simulink model "msdMultipleBuildingSoln"  (R2020b)
settings: Solver=VariableStepAuto  StartTime=0.0  StopTime=200  RelTol=1e-6
undefined symbols (not defined in the file): c, k, m, n, x_0, x_dot_0
settings Model: Creator=Rocksmithed  LastModifiedBy=Rocksmithed
settings DataIOCC: SaveFormat=Array
settings HardwareCC: TargetBitPerPointer=64  TargetBitPerSizeT=64  TargetBitPerPtrDiffT=64  TargetLongLongMode=on  TargetIntDivRoundTo=Zero  TargetEndianess=LittleEndian  TargetWordSize=64  TargetHWDeviceType=MATLAB Host  ProdEqTarget=off
settings RTWCC: Description=Rapid Simulation Target  SystemTargetFile=rsim.tlc  TemplateMakefile=rsim_default_tmf
settings RSimTargetCC: TargetLangStandard=C99 (ISO)

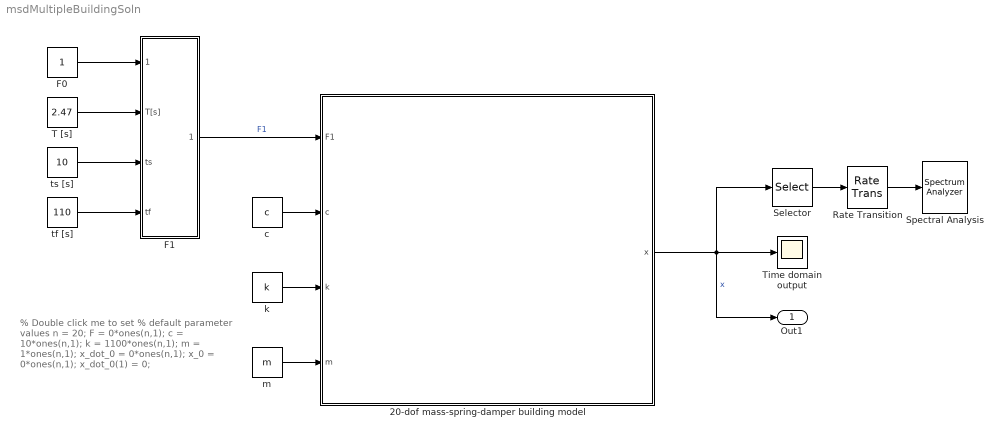
== system msdMultipleBuildingSoln ==
  note: % Double click me to set
      | % default parameter values
      | n = 20;
      | F = 0*ones(n,1);
      | c = 10*ones(n,1);
      | k = 1100*ones(n,1);
      | m = 1*ones(n,1);
      | x_dot_0 = 0*ones(n,1);
      | x_0 = 0*ones(n,1);
      | x_dot_0(1) = 0;
  20-dof mass-spring-damper building model : Subsystem  mask{x0_mask=x_0, x_dot_0_mask=x_dot_0}
      mask prompts: x0_mask "x0"; x_dot_0_mask "x_dot_0"
      mask Display: image('$imagefile'); % Use "Edit Image" on toolstrip to change.
  F0 : Constant
  F1 : Subsystem
  Rate Transition : RateTransition  OutPortSampleTime=0.05
  Selector : Selector  InputPortWidth=n  IndexOptions=Index vector (dialog)  Indices=20  OutputSizes=1
  Spectral Analysis : SpectrumAnalyzer
  T [s] : Constant  Value=2.47
  Time domain output : Scope
  c : Constant  Value=c
  k : Constant  Value=k
  m : Constant  Value=m
  tf [s] : Constant  Value=110
  ts [s] : Constant  Value=10
  Out1 : Outport
  wires:
  Selector/1 -> Rate Transition/1
  Rate Transition/1 -> Spectral Analysis/1
  20-dof mass-spring-damper building model/1(x) -> Selector/1, Out1/1, Time domain output/1  "x"
  c/1 -> 20-dof mass-spring-damper building model/2(c)
  k/1 -> 20-dof mass-spring-damper building model/3(k)
  m/1 -> 20-dof mass-spring-damper building model/4(m)
  tf [s]/1 -> F1/4(tf)
  T [s]/1 -> F1/2(T[s])
  ts [s]/1 -> F1/3(ts)
  F0/1 -> F1/1(F0 [N])
  F1/1(Out1) -> 20-dof mass-spring-damper building model/1(F1)  "F1"

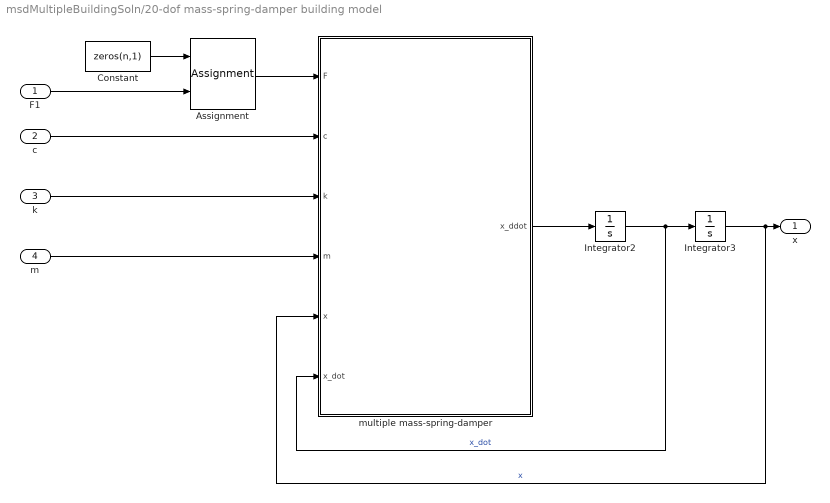
== system msdMultipleBuildingSoln/20-dof mass-spring-damper building model ==
  F1 : Inport
  c : Inport  Port=2
  k : Inport  Port=3
  m : Inport  Port=4
  Assignment : Assignment  DiagnosticForDimensions=Warning  IndexOptions=Index vector (dialog)  Indices=1  OutputSizes=1
  Constant : Constant  Value=zeros(n,1)
  Integrator2 : Integrator  InitialCondition=x_dot_0_mask
  Integrator3 : Integrator  InitialCondition=x0_mask
  multiple mass-spring-damper : MATLAB Function  TreatAsAtomicUnit=on
  x : Outport
  wires:
  k/1 -> multiple mass-spring-damper/3(k)
  Integrator2/1 -> multiple mass-spring-damper/6(x_dot), Integrator3/1  "x_dot"
  Integrator3/1 -> multiple mass-spring-damper/5(x), x/1  "x"
  multiple mass-spring-damper/1(x_ddot) -> Integrator2/1
  c/1 -> multiple mass-spring-damper/2(c)
  m/1 -> multiple mass-spring-damper/4(m)
  F1/1 -> Assignment/2
  Constant/1 -> Assignment/1
  Assignment/1 -> multiple mass-spring-damper/1(F)

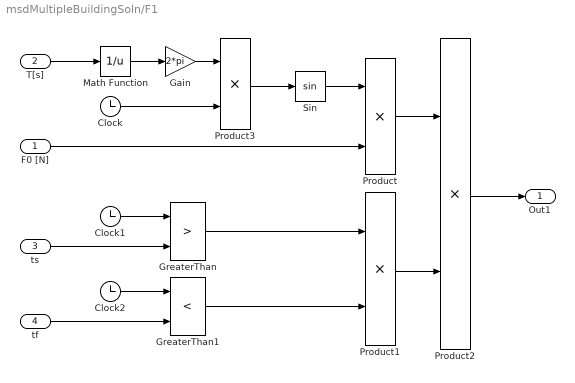
== system msdMultipleBuildingSoln/F1 ==
  F0 [N] : Inport
  T[s] : Inport  Port=2
  ts : Inport  Port=3
  tf : Inport  Port=4
  Clock : Clock
  Clock1 : Clock
  Clock2 : Clock
  Gain : Gain  Gain=2*pi
  GreaterThan : RelationalOperator  Operator=>  OutDataTypeStr=boolean  RndMeth=Simplest
  GreaterThan1 : RelationalOperator  Operator=<  OutDataTypeStr=boolean  RndMeth=Simplest
  Math Function : Math  Operator=reciprocal  SaturateOnIntegerOverflow=on
  Product{,1..3} (4 alike) : Product
  Sin : Trigonometry
  Out1 : Outport
  wires:
  GreaterThan/1 -> Product1/1
  GreaterThan1/1 -> Product1/2
  Product2/1 -> Out1/1
  Product/1 -> Product2/1
  Product1/1 -> Product2/2
  Math Function/1 -> Gain/1
  Gain/1 -> Product3/1
  Clock/1 -> Product3/2
  Product3/1 -> Sin/1
  Sin/1 -> Product/1
  F0 [N]/1 -> Product/2
  T[s]/1 -> Math Function/1
  Clock1/1 -> GreaterThan/1
  ts/1 -> GreaterThan/2
  Clock2/1 -> GreaterThan1/1
  tf/1 -> GreaterThan1/2

== matlab function msdMultipleBuildingSoln/20-dof mass-spring-damper building model/multiple mass-spring-damper ==
  data: F input; x_ddot output; c input; k input; m input; x input; x_dot input
function x_ddot = multipleMassSpringDamper(F, c, k, m, x, x_dot)
%#codegen

n = 20;

x_ddot = zeros(n,1);

x_ddot(1) = -(-F(1)+c(1).*x_dot(1)+k(1).*x(1)+c(2).*(x_dot(1)-x_dot(2))+k(2).*(x(1)-x(2)))./m(1);
if (n > 2)
    x_ddot(2:n-1) = F(2:n-1) + k(3:n).*( x(3:n) - x(2:n-1) ) + c(3:n).*( x_dot(3:n) - x_dot(2:n-1) )...
                             - k(2:n-1).*( x(2:n-1) - x(1:n-2) ) - c(2:n-1).*( x_dot(2:n-1) - x_dot(1:n-2) );
end
x_ddot(n) = (F(n)-c(n).*(x_dot(n)-x_dot(n-1))-k(n).*(x(n)-x(n-1)))./m(n) ;
